simulink model "matrix_mult_test"  (R2016b)
settings: Solver=ode4  StartTime=0.0  StopTime=400  FixedStep=0.001  RelTol=1e-3
undefined symbols (not defined in the file): v, w
settings Model: Creator=Kristian  LastModifiedBy=Kristian

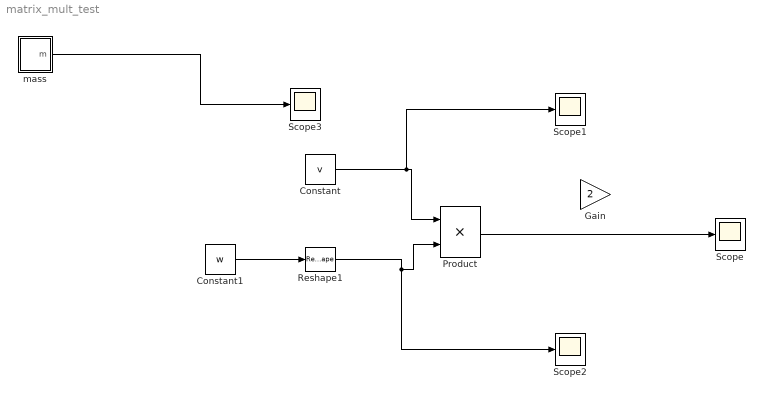
== system matrix_mult_test ==
  Constant : Constant  Value=v
  Constant1 : Constant  Value=w
  Gain : Gain  Gain=2
  Product : Product
  Reshape1 : Reshape  OutputDimensionality=Column vector (2-D)
  Scope{,1..3} (4 alike) : Scope
  "mass " : Subsystem
  wires:
  Constant/1 -> Scope1/1, Product/1
  Constant1/1 -> Reshape1/1
  Product/1 -> Scope/1
  Reshape1/1 -> Scope2/1, Product/2
  "mass "/1(m) -> Scope3/1

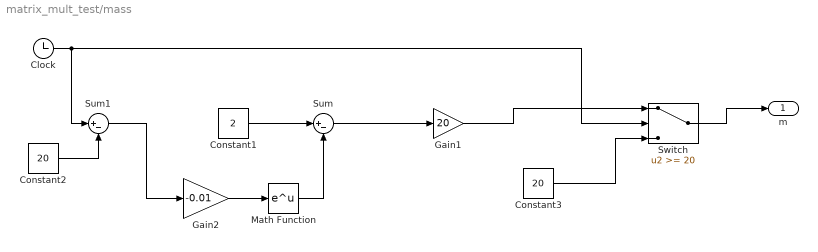
== system matrix_mult_test/mass  ==
  Clock : Clock
  Constant1 : Constant  Value=2
  Constant2 : Constant  Value=20
  Constant3 : Constant  Value=20
  Gain1 : Gain  Gain=20
  Gain2 : Gain  Gain=-0.01
  Math Function : Math  SaturateOnIntegerOverflow=on
  Sum : Sum  Inputs=|+-
  Sum1 : Sum  Inputs=|+-
  Switch : Switch  Threshold=20
  m : Outport
  wires:
  Clock/1 -> Sum1/1, Switch/2
  Switch/1 -> m/1
  Constant3/1 -> Switch/3
  Sum/1 -> Gain1/1
  Math Function/1 -> Sum/2
  Constant1/1 -> Sum/1
  Gain1/1 -> Switch/1
  Gain2/1 -> Math Function/1
  Constant2/1 -> Sum1/2
  Sum1/1 -> Gain2/1
